simulink model "ControlCSMSW"  (R2013b)
settings: Solver=ode45  StartTime=0.0  StopTime=10.0  FixedStep=0.0001  RelTol=1e-3
values from neighbouring files (symbols this model uses):
  cP = 500    [GimbalParameters.m]
  cT = 500    [GimbalParameters.m]
  epsilonP = 0.001    [GimbalParameters.m]
  epsilonT = 0.001    [GimbalParameters.m]
  IPx = 0.00261671    [GimbalParameters.m]
  IPy = 0.00247003    [GimbalParameters.m]
  IPz = 0.00046644    [GimbalParameters.m]
  ITx = 0.00016769    [GimbalParameters.m]
  ITy = 0.00017817    [GimbalParameters.m]
  ITz = 0.00011559    [GimbalParameters.m]
  KPcf = 0.0036    [GimbalParameters.m]
  KPvf = 0.0052    [GimbalParameters.m]
  KTcf = 0.0036    [GimbalParameters.m]
  KTvf = 0.0052    [GimbalParameters.m]
  rhoP = 50    [GimbalParameters.m]
  rhoT = 70    [GimbalParameters.m]
settings Model: Creator=Carlos Isaac  LastModifiedBy=Carlos Isaac

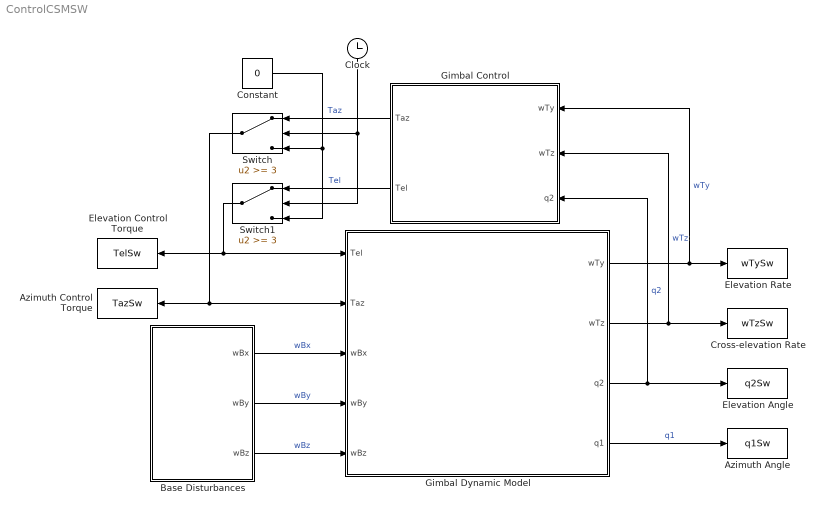
== system ControlCSMSW ==
  Azimuth Angle : ToWorkspace  VariableName=q1Sw  SampleTime=-1  SaveFormat=Timeseries
  Azimuth Control Torque : ToWorkspace  VariableName=TazSw  SampleTime=-1  SaveFormat=Timeseries
  Base Disturbances : Subsystem
  Clock : Clock
  Constant : Constant  Value=0
  Cross-elevation Rate : ToWorkspace  VariableName=wTzSw  SampleTime=-1  SaveFormat=Timeseries
  Elevation Angle : ToWorkspace  VariableName=q2Sw  SampleTime=-1  SaveFormat=Timeseries
  Elevation Control Torque : ToWorkspace  VariableName=TelSw  SampleTime=-1  SaveFormat=Timeseries
  Elevation Rate : ToWorkspace  VariableName=wTySw  SampleTime=-1  SaveFormat=Timeseries
  Gimbal Control : Subsystem
  Gimbal Dynamic Model : Subsystem
  Switch : Switch  Threshold=3
  Switch1 : Switch  Threshold=3
  wires:
  Base Disturbances/1(wBx) -> Gimbal Dynamic Model/3(wBx)  "wBx"
  Base Disturbances/2(wBy) -> Gimbal Dynamic Model/4(wBy)  "wBy"
  Base Disturbances/3(wBz) -> Gimbal Dynamic Model/5("wBz ")  "wBz"
  Switch1/1 -> Elevation Control Torque/1, Gimbal Dynamic Model/1(Tel)
  Switch/1 -> Azimuth Control Torque/1, Gimbal Dynamic Model/2(Taz)
  Clock/1 -> Switch/2, Switch1/2
  Gimbal Control/2(Tel) -> Switch1/1  "Tel"
  Gimbal Control/1(Taz) -> Switch/1  "Taz"
  Constant/1 -> Switch1/3, Switch/3
  Gimbal Dynamic Model/1(wTy) -> Elevation Rate/1, Gimbal Control/1(wTy)  "wTy"
  Gimbal Dynamic Model/2(wTz) -> Cross-elevation Rate/1, Gimbal Control/2(wTz)  "wTz"
  Gimbal Dynamic Model/3(q2) -> Elevation Angle/1, Gimbal Control/3(q2)  "q2"
  Gimbal Dynamic Model/4(q1) -> Azimuth Angle/1  "q1"

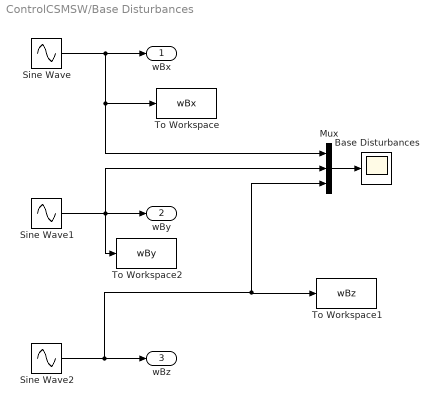
== system ControlCSMSW/Base Disturbances ==
  Base Disturbances : Scope
      settings: ShowLegends=on
  Mux : Mux  Inputs=3
  Sine Wave : Sin  Amplitude=1.5  Frequency=0.62831853  SampleTime=0
  Sine Wave1 : Sin  Amplitude=0.2  Frequency=1.88495559  SampleTime=0
  Sine Wave2 : Sin  Amplitude=0.8  Frequency=6.2831853  SampleTime=0
  To Workspace : ToWorkspace  VariableName=wBx  SampleTime=-1  SaveFormat=Timeseries
  To Workspace1 : ToWorkspace  VariableName=wBz  SampleTime=-1  SaveFormat=Timeseries
  To Workspace2 : ToWorkspace  VariableName=wBy  SampleTime=-1  SaveFormat=Timeseries
  wBx : Outport
  wBy : Outport  Port=2
  wBz : Outport  Port=3
  wires:
  Sine Wave/1 -> To Workspace/1, Mux/1, wBx/1
  Sine Wave1/1 -> To Workspace2/1, Mux/2, wBy/1
  Sine Wave2/1 -> To Workspace1/1, Mux/3, wBz/1
  Mux/1 -> Base Disturbances/1

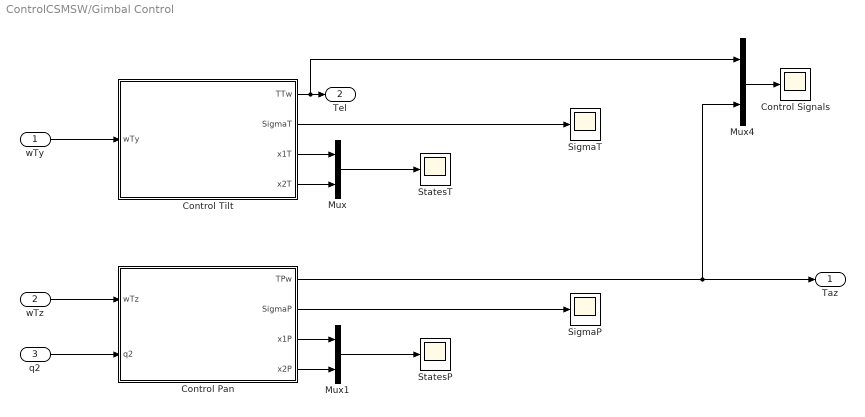
== system ControlCSMSW/Gimbal Control ==
  wTy : Inport
  wTz : Inport  Port=2
  q2 : Inport  Port=3
  Control Pan : Subsystem
  Control Signals : Scope
      settings: ShowLegends=on  SaveName=ScopeData6
  Control Tilt : Subsystem
  Mux : Mux  Inputs=2
  Mux1 : Mux  Inputs=2
  Mux4 : Mux  Inputs=2
  SigmaP : Scope
      settings: SaveName=ScopeData10
  SigmaT : Scope
      settings: SaveName=ScopeData8
  StatesP : Scope
      settings: SaveName=ScopeData11
  StatesT : Scope
      settings: SaveName=ScopeData9
  Taz : Outport
  Tel : Outport  Port=2
  wires:
  wTy/1 -> Control Tilt/1(wTy)
  Control Pan/1(TPw) -> Mux4/2, Taz/1
  wTz/1 -> Control Pan/1(wTz)
  Control Tilt/1(TTw) -> Mux4/1, Tel/1
  Control Tilt/2(SigmaT) -> SigmaT/1
  Control Tilt/4(x2T) -> Mux/2
  Control Tilt/3(x1T) -> Mux/1
  Mux/1 -> StatesT/1
  Mux4/1 -> Control Signals/1
  Control Pan/2(SigmaP) -> SigmaP/1
  Control Pan/4(x2P) -> Mux1/2
  Control Pan/3(x1P) -> Mux1/1
  Mux1/1 -> StatesP/1
  q2/1 -> Control Pan/2(q2)

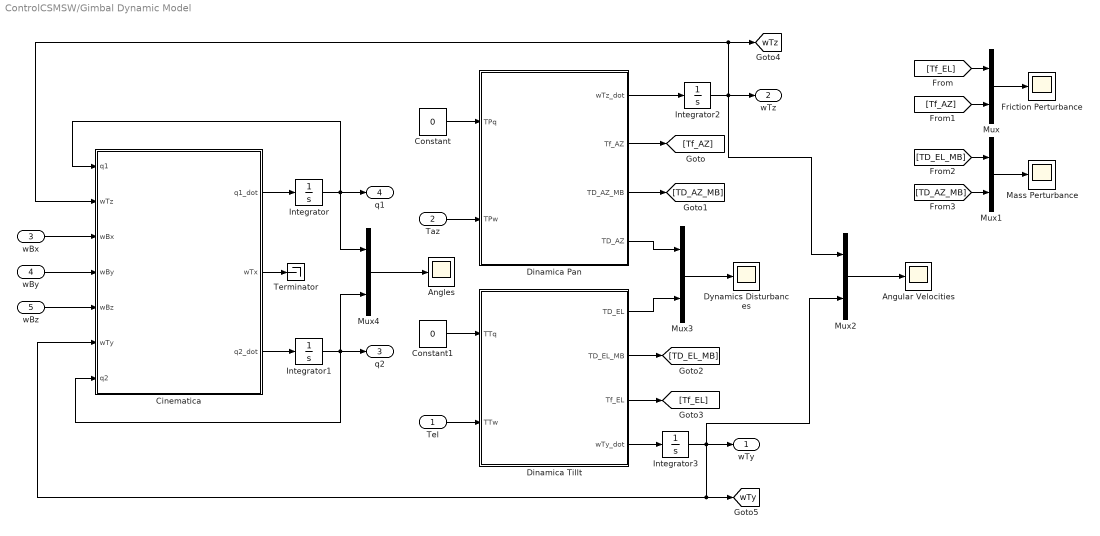
== system ControlCSMSW/Gimbal Dynamic Model ==
  Tel : Inport
  Taz : Inport  Port=2
  wBx : Inport  Port=3
  wBy : Inport  Port=4
  "wBz " : Inport  Port=5
  Angles : Scope
      settings: SaveName=ScopeData2
  Angular Velocities : Scope
      settings: ShowLegends=on
  Cinematica : Subsystem
  Constant : Constant  Value=0
  Constant1 : Constant  Value=0
  Dinamica Pan : Subsystem
  Dinamica Tillt : Subsystem
  Dynamics Disturbances : Scope
      settings: SaveName=ScopeData3
  Friction Perturbance : Scope
      settings: SaveName=ScopeData4
  Integrator{,1..3} (4 alike) : Integrator
  Mass Perturbance : Scope
      settings: SaveName=ScopeData5
  Mux{,1..4} (5 alike) : Mux  Inputs=2
  Terminator : Terminator
  wTy : Outport
  wTz : Outport  Port=2
  q2 : Outport  Port=3
  q1 : Outport  Port=4
  tag scope: wTy=global, wTz=global
  wires:
  Cinematica/3(q2_dot) -> Integrator1/1
  Integrator/1 -> q1/1, Mux4/1, Cinematica/1(q1)
  Integrator1/1 -> Mux4/2, Cinematica/7(q2), q2/1
  Dinamica Pan/1(wTz_dot) -> Integrator2/1
  Integrator2/1 -> Mux2/1, wTz/1, Cinematica/2(wTz), [wTz]
  Integrator3/1 -> wTy/1, Mux2/2, Cinematica/6(wTy), [wTy]
  Cinematica/2(wTx) -> Terminator/1
  Cinematica/1(q1_dot) -> Integrator/1
  "wBz "/1 -> Cinematica/5(wBz)
  wBy/1 -> Cinematica/4(wBy)
  wBx/1 -> Cinematica/3(wBx)
  Constant/1 -> Dinamica Pan/1(TPq)
  Taz/1 -> Dinamica Pan/2(TPw)
  Dinamica Tillt/4(wTy_dot) -> Integrator3/1
  Dinamica Pan/2(Tf_AZ) -> [Tf_AZ]
  Dinamica Pan/3(TD_AZ_MB) -> [TD_AZ_MB]
  Dinamica Tillt/2(TD_EL_MB) -> [TD_EL_MB]
  Dinamica Tillt/3(Tf_EL) -> [Tf_EL]
  [Tf_EL] -> Mux/1
  [Tf_AZ] -> Mux/2
  Mux/1 -> Friction Perturbance/1
  [TD_EL_MB] -> Mux1/1
  [TD_AZ_MB] -> Mux1/2
  Mux1/1 -> Mass Perturbance/1
  Tel/1 -> Dinamica Tillt/2(TTw)
  Constant1/1 -> Dinamica Tillt/1(TTq)
  Mux3/1 -> Dynamics Disturbances/1
  Dinamica Pan/4(TD_AZ) -> Mux3/1
  Dinamica Tillt/1(TD_EL) -> Mux3/2
  Mux4/1 -> Angles/1
  Mux2/1 -> Angular Velocities/1

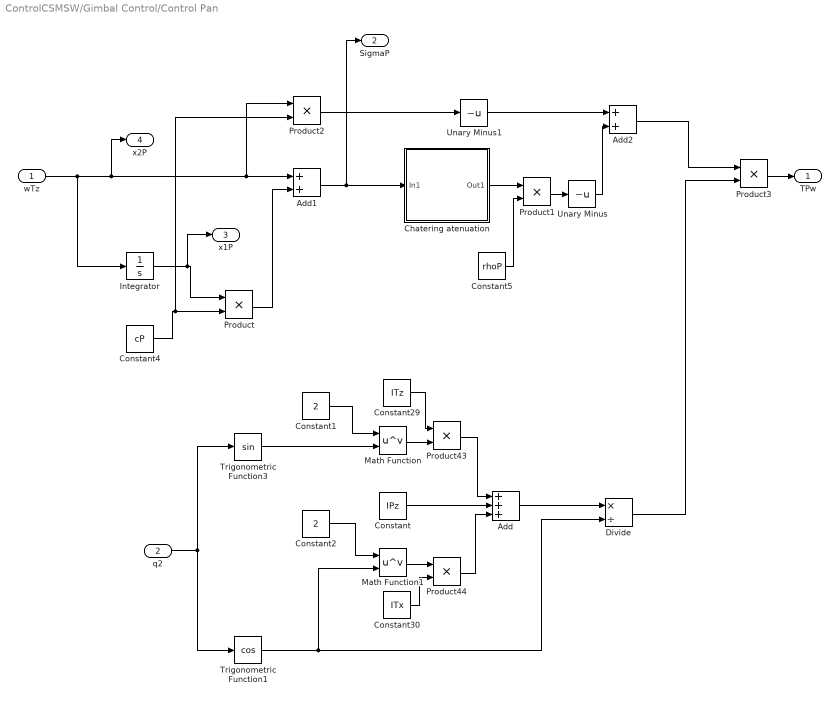
== system ControlCSMSW/Gimbal Control/Control Pan ==
  wTz : Inport
  q2 : Inport  Port=2
  Add : Sum  Inputs=+++
  Add1 : Sum
  Add2 : Sum
  Chatering atenuation : Subsystem
  Constant : Constant  Value=IPz
  Constant1 : Constant  Value=2
  Constant2 : Constant  Value=2
  Constant29 : Constant  Value=ITz
  Constant30 : Constant  Value=ITx
  Constant4 : Constant  Value=cP
  Constant5 : Constant  Value=rhoP
  Divide : Product  Inputs=*/
  Integrator : Integrator
  Math Function : Math  Operator=pow  SaturateOnIntegerOverflow=on
  Math Function1 : Math  Operator=pow  SaturateOnIntegerOverflow=on
  Product{,1..3,43..44} (6 alike) : Product
  Trigonometric Function1 : Trigonometry  Operator=cos
  Trigonometric Function3 : Trigonometry
  Unary Minus : UnaryMinus
  Unary Minus1 : UnaryMinus
  TPw : Outport
  SigmaP : Outport  Port=2
  x1P : Outport  Port=3
  x2P : Outport  Port=4
  wires:
  wTz/1 -> Integrator/1, x2P/1, Product2/1, Add1/1
  Integrator/1 -> x1P/1, Product/1
  Constant4/1 -> Product2/2, Product/2
  Product/1 -> Add1/2
  Constant5/1 -> Product1/2
  Product1/1 -> Unary Minus/1
  Product2/1 -> Unary Minus1/1
  Unary Minus1/1 -> Add2/1
  Unary Minus/1 -> Add2/2
  Chatering atenuation/1(Out1) -> Product1/1
  Add1/1 -> SigmaP/1, Chatering atenuation/1(In1)
  Constant1/1 -> Math Function/1
  Trigonometric Function3/1 -> Math Function/2
  Constant2/1 -> Math Function1/1
  Trigonometric Function1/1 -> Math Function1/2, Divide/2
  Constant/1 -> Add/2
  Add/1 -> Divide/1
  q2/1 -> Trigonometric Function1/1, Trigonometric Function3/1
  Divide/1 -> Product3/2
  Constant29/1 -> Product43/1
  Math Function/1 -> Product43/2
  Product43/1 -> Add/1
  Constant30/1 -> Product44/2
  Math Function1/1 -> Product44/1
  Product44/1 -> Add/3
  Product3/1 -> TPw/1
  Add2/1 -> Product3/1

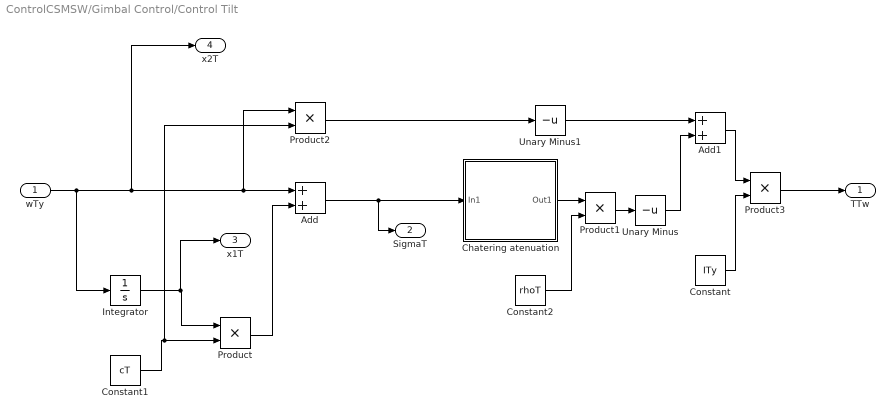
== system ControlCSMSW/Gimbal Control/Control Tilt ==
  wTy : Inport
  Add : Sum
  Add1 : Sum
  Chatering atenuation : Subsystem
  Constant : Constant  Value=ITy
  Constant1 : Constant  Value=cT
  Constant2 : Constant  Value=rhoT
  Integrator : Integrator
  Product{,1..3} (4 alike) : Product
  Unary Minus : UnaryMinus
  Unary Minus1 : UnaryMinus
  TTw : Outport
  SigmaT : Outport  Port=2
  x1T : Outport  Port=3
  x2T : Outport  Port=4
  wires:
  wTy/1 -> Integrator/1, x2T/1, Product2/1, Add/1
  Integrator/1 -> x1T/1, Product/1
  Constant1/1 -> Product2/2, Product/2
  Product/1 -> Add/2
  Constant2/1 -> Product1/2
  Product1/1 -> Unary Minus/1
  Product2/1 -> Unary Minus1/1
  Unary Minus1/1 -> Add1/1
  Unary Minus/1 -> Add1/2
  Add1/1 -> Product3/1
  Constant/1 -> Product3/2
  Product3/1 -> TTw/1
  Chatering atenuation/1(Out1) -> Product1/1
  Add/1 -> SigmaT/1, Chatering atenuation/1(In1)

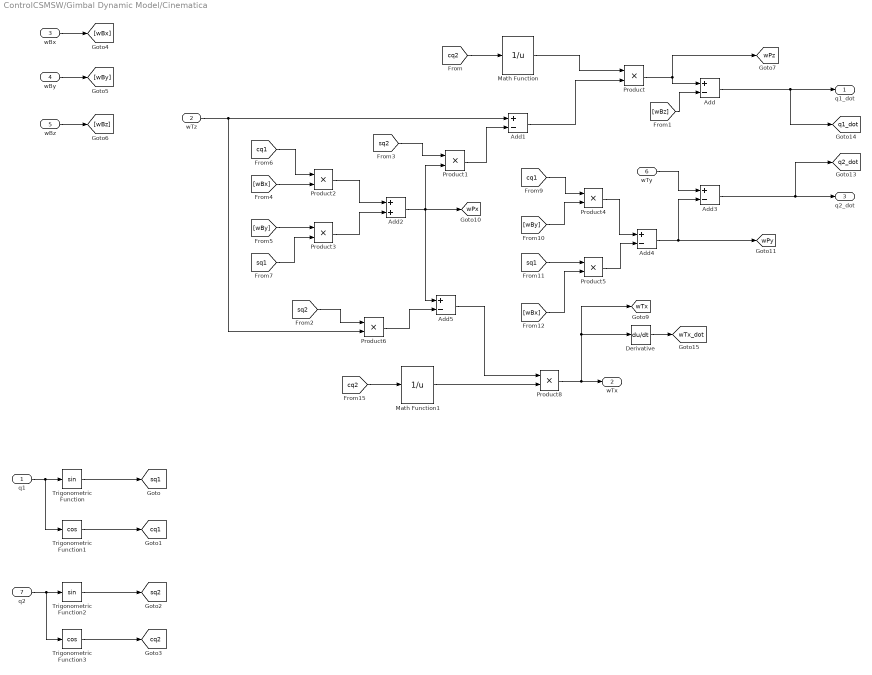
== system ControlCSMSW/Gimbal Dynamic Model/Cinematica ==
  q1 : Inport
  wTz : Inport  Port=2
  wBx : Inport  Port=3
  wBy : Inport  Port=4
  wBz : Inport  Port=5
  wTy : Inport  Port=6
  q2 : Inport  Port=7
  Add{,1,3..5} (5 alike) : Sum  Inputs=+-
  Add2 : Sum
  Derivative : Derivative
  Math Function : Math  Operator=reciprocal  SaturateOnIntegerOverflow=on
  Math Function1 : Math  Operator=reciprocal  SaturateOnIntegerOverflow=on
  Product{,1..6,8} (8 alike) : Product
  Trigonometric Function : Trigonometry
  Trigonometric Function1 : Trigonometry  Operator=cos
  Trigonometric Function2 : Trigonometry
  Trigonometric Function3 : Trigonometry  Operator=cos
  q1_dot : Outport
  wTx : Outport  Port=2
  q2_dot : Outport  Port=3
  tag scope: cq1=global, cq2=global, q1_dot=global, q2_dot=global, sq1=global, sq2=global, wPx=global, wPy=global, wPz=global, wTx=global, wTx_dot=global
  wires:
  Trigonometric Function/1 -> [sq1]
  Trigonometric Function1/1 -> [cq1]
  Trigonometric Function2/1 -> [sq2]
  Trigonometric Function3/1 -> [cq2]
  q1/1 -> Trigonometric Function1/1, Trigonometric Function/1
  q2/1 -> Trigonometric Function3/1, Trigonometric Function2/1
  wBx/1 -> [wBx]
  wBy/1 -> [wBy]
  wBz/1 -> [wBz]
  [cq2] -> Math Function/1
  Math Function/1 -> Product/1
  Product/1 -> [wPz], Add/1
  Add/1 -> [q1_dot], q1_dot/1
  [wBz] -> Add/2
  Add1/1 -> Product/2
  Product1/1 -> Add1/2
  [sq2] -> Product1/1
  Add2/1 -> Add5/1, [wPx], Product1/2
  Product2/1 -> Add2/1
  Product3/1 -> Add2/2
  [wBx] -> Product2/2
  [wBy] -> Product3/1
  [cq1] -> Product2/1
  [sq1] -> Product3/2
  Add3/1 -> [q2_dot], q2_dot/1
  wTy/1 -> Add3/1
  Add4/1 -> [wPy], Add3/2
  Product4/1 -> Add4/1
  [cq1] -> Product4/1
  [wBy] -> Product4/2
  Product5/1 -> Add4/2
  [sq1] -> Product5/1
  [wBx] -> Product5/2
  wTz/1 -> Product6/2, Add1/1
  Derivative/1 -> [wTx_dot]
  [cq2] -> Math Function1/1
  Product8/1 -> wTx/1, [wTx], Derivative/1
  Math Function1/1 -> Product8/2
  Add5/1 -> Product8/1
  [sq2] -> Product6/1
  Product6/1 -> Add5/2

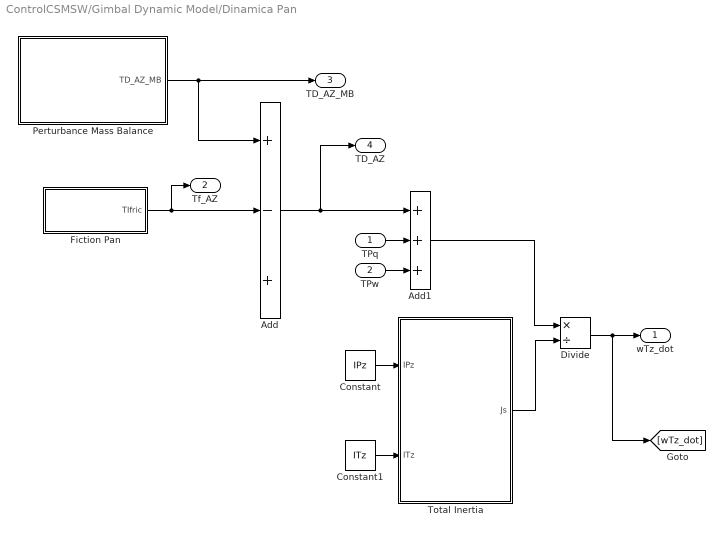
== system ControlCSMSW/Gimbal Dynamic Model/Dinamica Pan ==
  TPq : Inport
  TPw : Inport  Port=2
  Add : Sum  Inputs=+-+
  Add1 : Sum  Inputs=+++
  Constant : Constant  Value=IPz
  Constant1 : Constant  Value=ITz
  Divide : Product  Inputs=*/
  Fiction Pan : Subsystem
  Perturbance Mass Balance : Subsystem
  Total Inertia : Subsystem
  wTz_dot : Outport
  Tf_AZ : Outport  Port=2
  TD_AZ_MB : Outport  Port=3
  TD_AZ : Outport  Port=4
  wires:
  Fiction Pan/1(TIfric) -> Tf_AZ/1, Add/2
  Divide/1 -> [wTz_dot], wTz_dot/1
  Total Inertia/1(Js) -> Divide/2
  Perturbance Mass Balance/1(TD_AZ_MB) -> Add/1, TD_AZ_MB/1
  Constant/1 -> Total Inertia/1(IPz)
  Constant1/1 -> Total Inertia/2(ITz)
  Add1/1 -> Divide/1
  Add/1 -> TD_AZ/1, Add1/1
  TPw/1 -> Add1/3
  TPq/1 -> Add1/2

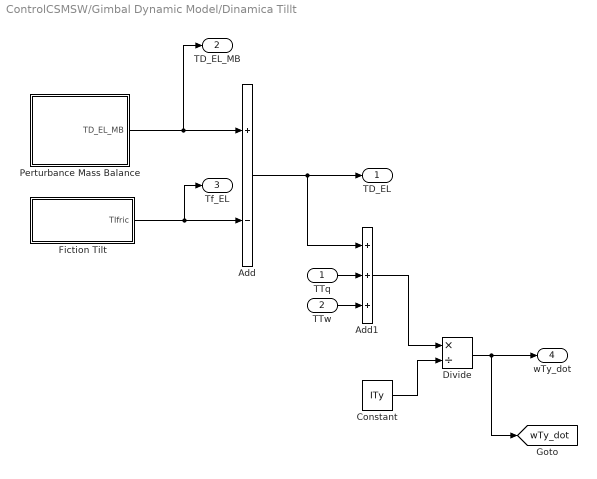
== system ControlCSMSW/Gimbal Dynamic Model/Dinamica Tillt ==
  TTq : Inport
  TTw : Inport  Port=2
  Add : Sum  Inputs=+-
  Add1 : Sum  Inputs=+++
  Constant : Constant  Value=ITy
  Divide : Product  Inputs=*/
  Fiction Tilt : Subsystem
  Perturbance Mass Balance : Subsystem
  TD_EL : Outport
  TD_EL_MB : Outport  Port=2
  Tf_EL : Outport  Port=3
  wTy_dot : Outport  Port=4
  tag scope: wTy_dot=global
  wires:
  Perturbance Mass Balance/1(TD_EL_MB) -> TD_EL_MB/1, Add/1
  Fiction Tilt/1(TIfric) -> Tf_EL/1, Add/2
  Constant/1 -> Divide/2
  Divide/1 -> [wTy_dot], wTy_dot/1
  Add1/1 -> Divide/1
  Add/1 -> TD_EL/1, Add1/1
  TTq/1 -> Add1/2
  TTw/1 -> Add1/3

== system ControlCSMSW/Gimbal Control/Control Pan/Chatering atenuation ==
  In1 : Inport
  Abs : Abs
  Add : Sum
  Constant : Constant  Value=epsilonP
  Divide : Product  Inputs=*/
  Out1 : Outport
  wires:
  In1/1 -> Abs/1, Divide/1
  Abs/1 -> Add/1
  Add/1 -> Divide/2
  Divide/1 -> Out1/1
  Constant/1 -> Add/2

== system ControlCSMSW/Gimbal Control/Control Tilt/Chatering atenuation ==
  In1 : Inport
  Abs : Abs
  Add : Sum
  Constant : Constant  Value=epsilonT
  Divide : Product  Inputs=*/
  Out1 : Outport
  wires:
  In1/1 -> Abs/1, Divide/1
  Abs/1 -> Add/1
  Add/1 -> Divide/2
  Divide/1 -> Out1/1
  Constant/1 -> Add/2

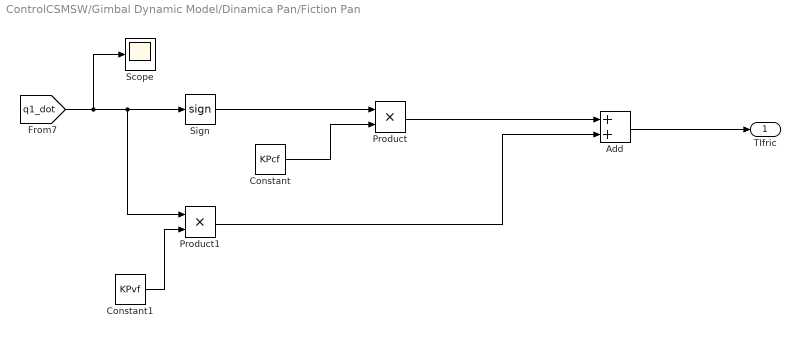
== system ControlCSMSW/Gimbal Dynamic Model/Dinamica Pan/Fiction Pan ==
  Add : Sum
  Constant : Constant  Value=KPcf
  Constant1 : Constant  Value=KPvf
  Product : Product
  Product1 : Product
  Scope : Scope
      settings: SaveName=ScopeData7
  Sign : Signum  ZeroCross=off
  TIfric : Outport
  wires:
  [q1_dot] -> Scope/1, Product1/1, Sign/1
  Sign/1 -> Product/1
  Constant/1 -> Product/2
  Constant1/1 -> Product1/2
  Product/1 -> Add/1
  Product1/1 -> Add/2
  Add/1 -> TIfric/1

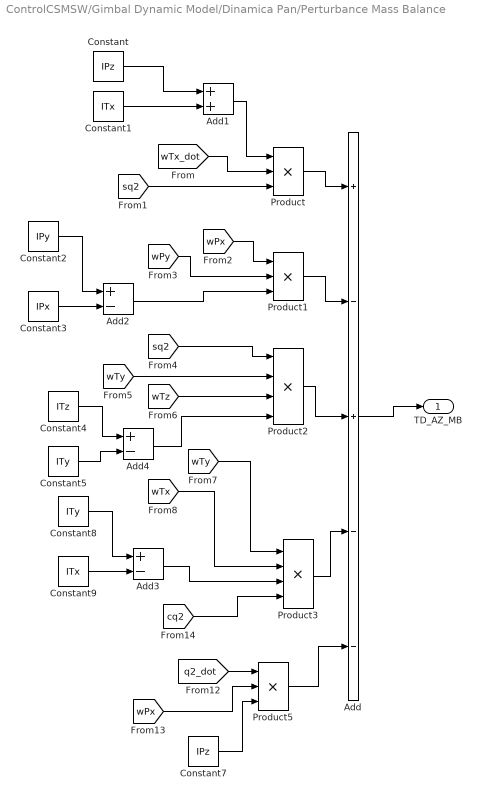
== system ControlCSMSW/Gimbal Dynamic Model/Dinamica Pan/Perturbance Mass Balance ==
  Add : Sum  Inputs=+-+--
  Add1 : Sum
  Add2 : Sum  Inputs=+-
  Add3 : Sum  Inputs=+-
  Add4 : Sum  Inputs=+-
  Constant : Constant  Value=IPz
  Constant1 : Constant  Value=ITx
  Constant2 : Constant  Value=IPy
  Constant3 : Constant  Value=IPx
  Constant4 : Constant  Value=ITz
  Constant5 : Constant  Value=ITy
  Constant7 : Constant  Value=IPz
  Constant8 : Constant  Value=ITy
  Constant9 : Constant  Value=ITx
  Product : Product  Inputs=3
  Product1 : Product  Inputs=3
  Product2 : Product  Inputs=4
  Product3 : Product  Inputs=4
  Product5 : Product  Inputs=3
  TD_AZ_MB : Outport
  wires:
  Add/1 -> TD_AZ_MB/1
  Product/1 -> Add/1
  Constant/1 -> Add1/1
  Constant1/1 -> Add1/2
  Add1/1 -> Product/1
  [wTx_dot] -> Product/2
  [sq2] -> Product/3
  Product1/1 -> Add/2
  [wPx] -> Product1/1
  [wPy] -> Product1/2
  Add2/1 -> Product1/3
  Constant2/1 -> Add2/1
  Constant3/1 -> Add2/2
  Product2/1 -> Add/3
  [sq2] -> Product2/1
  [wTz] -> Product2/3
  [wTy] -> Product2/2
  Product3/1 -> Add/4
  [wTy] -> Product3/1
  [wTx] -> Product3/2
  [q2_dot] -> Product5/1
  [wPx] -> Product5/2
  Constant7/1 -> Product5/3
  Product5/1 -> Add/5
  Constant8/1 -> Add3/1
  Constant9/1 -> Add3/2
  Add3/1 -> Product3/3
  [cq2] -> Product3/4
  Add4/1 -> Product2/4
  Constant4/1 -> Add4/1
  Constant5/1 -> Add4/2

== system ControlCSMSW/Gimbal Dynamic Model/Dinamica Pan/Total Inertia ==
  IPz : Inport
  ITz : Inport  Port=2
  Add : Sum
  Product : Product
  Js : Outport
  wires:
  IPz/1 -> Add/1
  ITz/1 -> Add/2
  Add/1 -> Product/2
  Product/1 -> Js/1
  [cq2] -> Product/1

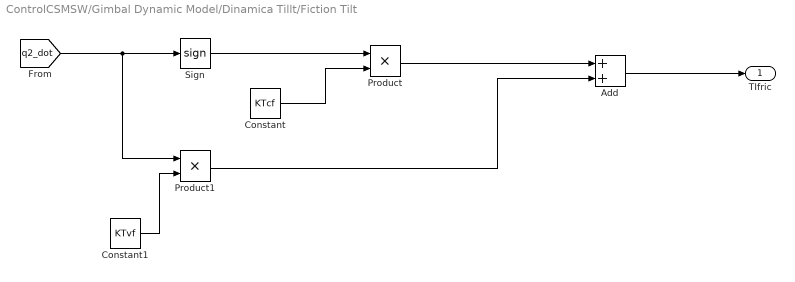
== system ControlCSMSW/Gimbal Dynamic Model/Dinamica Tillt/Fiction Tilt ==
  Add : Sum
  Constant : Constant  Value=KTcf
  Constant1 : Constant  Value=KTvf
  Product : Product
  Product1 : Product
  Sign : Signum  ZeroCross=off
  TIfric : Outport
  wires:
  [q2_dot] -> Product1/1, Sign/1
  Sign/1 -> Product/1
  Constant/1 -> Product/2
  Constant1/1 -> Product1/2
  Product/1 -> Add/1
  Product1/1 -> Add/2
  Add/1 -> TIfric/1

== system ControlCSMSW/Gimbal Dynamic Model/Dinamica Tillt/Perturbance Mass Balance ==
  Add : Sum  Inputs=+-
  Constant : Constant  Value=ITz
  Constant1 : Constant  Value=ITx
  Product : Product
  Product1 : Product
  TD_EL_MB : Outport
  wires:
  Constant/1 -> Add/1
  Constant1/1 -> Add/2
  Product/1 -> Product1/1
  Add/1 -> Product1/2
  Product1/1 -> TD_EL_MB/1
  [wTx] -> Product/1
  [wTz] -> Product/2
